simulink model "HANcoder_E407_DYS_MP"  (R2018b)
settings: Solver=FixedStepDiscrete  StartTime=0.0  StopTime=1  FixedStep=0.01  RelTol=1e-3
PreLoadFcn:
  | librarySetup
  | eval([bdroot,'_startup']) %Calling [modelName]_startup.m
values from neighbouring files (symbols this model uses):
  basic_cycle_duration_bc0 = TM_Reset_Board   + COMP_duration    (= 212)    [HANcoder_E407_DYS_MP_startup.m]
  basic_cycle_duration_bc1 = basic_cycle_duration_bc0    (= 212)    [HANcoder_E407_DYS_MP_startup.m]
  comm_delay_estimation1 = round(comm_delay_measured1*hardware_granularity/frequency_IRQ)    [HANcoder_E407_DYS_MP_startup.m]
  comm_delay_estimation2 = round(comm_delay_measured2*hardware_granularity/frequency_IRQ)    [HANcoder_E407_DYS_MP_startup.m]
  COMM_Phase1 = Simulink.Parameter    [HANcoder_E407_DYS_MP_startup.m]
  COMM_Phase2 = Simulink.Parameter    [HANcoder_E407_DYS_MP_startup.m]
  frequency_IRQ = 500    [HANcoder_E407_DYS_MP_startup.m]
  HantuneAngleSp = Simulink.Parameter    [HANcoder_E407_DYS_MP_startup.m]
  idle_time_init = basic_cycle_duration_bc0 + basic_cycle_duration_bc1    (= 424)    [HANcoder_E407_DYS_MP_startup.m]
  matrix_rows = 2    [HANcoder_E407_DYS_MP_startup.m]
  positionD = Simulink.Parameter    [HANcoder_E407_DYS_MP_startup.m]
  positionI = Simulink.Parameter    [HANcoder_E407_DYS_MP_startup.m]
  positionP = Simulink.Parameter    [HANcoder_E407_DYS_MP_startup.m]
undefined symbols (not defined in the file or in its folder): A1, CON2, CON4, D13, Dposition, Iposition, Pposition
libraries: HANcoder_STM32_Target x33, dspswit3 x16, simulink x2, simulink_extras x2, dspstat3 x1
(part 9 of 10)

== system HANcoder_E407_DYS_MP/HANcoder STM32 Target - E407-STM32 algorithm/4.TTA Can System/4.3 TTA System/4.3.3 Matrix Cycle Manager/4.3.3.1 Controller Matrix Cycle Truck Boards 1 2 and 3/4.3.3.1.2 controller basic cycle 0.2/Receive Truck 2 Board 2 Calc Steering Angle/Receive can message/CAN receive2 ==
  In1 : Inport
  Enabled Subsystem : Subsystem  TreatAsAtomicUnit=on
  S-Function : M-S-Function  FunctionName=sfcn_can_receive  Parameters=tsamp, canBus, outputNumber, dataType, byteOrder
  Term{3..9} (7 alike) : Terminator
  Out1 : Outport
  Out2 : Outport  Port=2
  wires:
  S-Function/9 -> Enabled Subsystem/8(In8)
  S-Function/4 -> Enabled Subsystem/3(In3)
  S-Function/5 -> Enabled Subsystem/4(In4)
  S-Function/8 -> Enabled Subsystem/7(In7)
  S-Function/7 -> Enabled Subsystem/6(In6)
  S-Function/6 -> Enabled Subsystem/5(In5)
  Enabled Subsystem/8(Out8) -> Term9/1
  Enabled Subsystem/7(Out7) -> Term8/1
  Enabled Subsystem/6(Out6) -> Term7/1
  Enabled Subsystem/5(Out5) -> Term6/1
  Enabled Subsystem/4(Out4) -> Term5/1
  Enabled Subsystem/3(Out3) -> Term4/1
  Enabled Subsystem/2(Out2) -> Term3/1
  Enabled Subsystem/1(Out1) -> Out2/1
  S-Function/3 -> Enabled Subsystem/2(In2)
  S-Function/2 -> Enabled Subsystem/1(In1)
  S-Function/1 -> Out1/1, Enabled Subsystem/Enable
  In1/1 -> S-Function/1

== system HANcoder_E407_DYS_MP/HANcoder STM32 Target - E407-STM32 algorithm/4.TTA Can System/4.3 TTA System/4.3.3 Matrix Cycle Manager/4.3.3.1 Controller Matrix Cycle Truck Boards 1 2 and 3/4.3.3.1.2 controller basic cycle 0.2/Receive Truck 3 Board 3 Calc Steering Angle/Receive can message/CAN receive ==
  In1 : Inport
  Enabled Subsystem : Subsystem  TreatAsAtomicUnit=on
  S-Function : M-S-Function  FunctionName=sfcn_can_receive  Parameters=tsamp, canBus, outputNumber, dataType, byteOrder
  Term{3..9} (7 alike) : Terminator
  Out1 : Outport
  Out2 : Outport  Port=2
  wires:
  S-Function/9 -> Enabled Subsystem/8(In8)
  S-Function/4 -> Enabled Subsystem/3(In3)
  S-Function/5 -> Enabled Subsystem/4(In4)
  S-Function/8 -> Enabled Subsystem/7(In7)
  S-Function/7 -> Enabled Subsystem/6(In6)
  S-Function/6 -> Enabled Subsystem/5(In5)
  Enabled Subsystem/8(Out8) -> Term9/1
  Enabled Subsystem/7(Out7) -> Term8/1
  Enabled Subsystem/6(Out6) -> Term7/1
  Enabled Subsystem/5(Out5) -> Term6/1
  Enabled Subsystem/4(Out4) -> Term5/1
  Enabled Subsystem/3(Out3) -> Term4/1
  Enabled Subsystem/2(Out2) -> Term3/1
  Enabled Subsystem/1(Out1) -> Out2/1
  S-Function/3 -> Enabled Subsystem/2(In2)
  S-Function/2 -> Enabled Subsystem/1(In1)
  S-Function/1 -> Out1/1, Enabled Subsystem/Enable
  In1/1 -> S-Function/1

== system HANcoder_E407_DYS_MP/HANcoder STM32 Target - E407-STM32 algorithm/4.TTA Can System/4.3 TTA System/4.3.3 Matrix Cycle Manager/4.3.3.1 Controller Matrix Cycle Truck Boards 1 2 and 3/4.3.3.1.2 controller basic cycle 0.2/Receive Truck 3 Board 3 Calc Steering Angle/Receive can message/CAN receive2 ==
  In1 : Inport
  Enabled Subsystem : Subsystem  TreatAsAtomicUnit=on
  S-Function : M-S-Function  FunctionName=sfcn_can_receive  Parameters=tsamp, canBus, outputNumber, dataType, byteOrder
  Term{3..9} (7 alike) : Terminator
  Out1 : Outport
  Out2 : Outport  Port=2
  wires:
  S-Function/9 -> Enabled Subsystem/8(In8)
  S-Function/4 -> Enabled Subsystem/3(In3)
  S-Function/5 -> Enabled Subsystem/4(In4)
  S-Function/8 -> Enabled Subsystem/7(In7)
  S-Function/7 -> Enabled Subsystem/6(In6)
  S-Function/6 -> Enabled Subsystem/5(In5)
  Enabled Subsystem/8(Out8) -> Term9/1
  Enabled Subsystem/7(Out7) -> Term8/1
  Enabled Subsystem/6(Out6) -> Term7/1
  Enabled Subsystem/5(Out5) -> Term6/1
  Enabled Subsystem/4(Out4) -> Term5/1
  Enabled Subsystem/3(Out3) -> Term4/1
  Enabled Subsystem/2(Out2) -> Term3/1
  Enabled Subsystem/1(Out1) -> Out2/1
  S-Function/3 -> Enabled Subsystem/2(In2)
  S-Function/2 -> Enabled Subsystem/1(In1)
  S-Function/1 -> Out1/1, Enabled Subsystem/Enable
  In1/1 -> S-Function/1

== system HANcoder_E407_DYS_MP/HANcoder STM32 Target - E407-STM32 algorithm/4.TTA Can System/4.3 TTA System/4.3.3 Matrix Cycle Manager/4.3.3.2 Controller Matrix Cycle_Board 4 and 5/controller basic cycle 0/Receive Timer can master message /Receive can message/CAN receive ==
  In1 : Inport
  Enabled Subsystem : Subsystem  TreatAsAtomicUnit=on
  S-Function : M-S-Function  FunctionName=sfcn_can_receive  Parameters=tsamp, canBus, outputNumber, dataType, byteOrder
  Term{3..9} (7 alike) : Terminator
  Out1 : Outport
  Out2 : Outport  Port=2
  wires:
  S-Function/9 -> Enabled Subsystem/8(In8)
  S-Function/4 -> Enabled Subsystem/3(In3)
  S-Function/5 -> Enabled Subsystem/4(In4)
  S-Function/8 -> Enabled Subsystem/7(In7)
  S-Function/7 -> Enabled Subsystem/6(In6)
  S-Function/6 -> Enabled Subsystem/5(In5)
  Enabled Subsystem/8(Out8) -> Term9/1
  Enabled Subsystem/7(Out7) -> Term8/1
  Enabled Subsystem/6(Out6) -> Term7/1
  Enabled Subsystem/5(Out5) -> Term6/1
  Enabled Subsystem/4(Out4) -> Term5/1
  Enabled Subsystem/3(Out3) -> Term4/1
  Enabled Subsystem/2(Out2) -> Term3/1
  Enabled Subsystem/1(Out1) -> Out2/1
  S-Function/3 -> Enabled Subsystem/2(In2)
  S-Function/2 -> Enabled Subsystem/1(In1)
  S-Function/1 -> Out1/1, Enabled Subsystem/Enable
  In1/1 -> S-Function/1

== system HANcoder_E407_DYS_MP/HANcoder STM32 Target - E407-STM32 algorithm/4.TTA Can System/4.3 TTA System/4.3.3 Matrix Cycle Manager/4.3.3.2 Controller Matrix Cycle_Board 4 and 5/controller basic cycle 0/Receive Timer can master message /Receive can message/CAN receive2 ==
  In1 : Inport
  Enabled Subsystem : Subsystem  TreatAsAtomicUnit=on
  S-Function : M-S-Function  FunctionName=sfcn_can_receive  Parameters=tsamp, canBus, outputNumber, dataType, byteOrder
  Term{3..9} (7 alike) : Terminator
  Out1 : Outport
  Out2 : Outport  Port=2
  wires:
  S-Function/9 -> Enabled Subsystem/8(In8)
  S-Function/4 -> Enabled Subsystem/3(In3)
  S-Function/5 -> Enabled Subsystem/4(In4)
  S-Function/8 -> Enabled Subsystem/7(In7)
  S-Function/7 -> Enabled Subsystem/6(In6)
  S-Function/6 -> Enabled Subsystem/5(In5)
  Enabled Subsystem/8(Out8) -> Term9/1
  Enabled Subsystem/7(Out7) -> Term8/1
  Enabled Subsystem/6(Out6) -> Term7/1
  Enabled Subsystem/5(Out5) -> Term6/1
  Enabled Subsystem/4(Out4) -> Term5/1
  Enabled Subsystem/3(Out3) -> Term4/1
  Enabled Subsystem/2(Out2) -> Term3/1
  Enabled Subsystem/1(Out1) -> Out2/1
  S-Function/3 -> Enabled Subsystem/2(In2)
  S-Function/2 -> Enabled Subsystem/1(In1)
  S-Function/1 -> Out1/1, Enabled Subsystem/Enable
  In1/1 -> S-Function/1

== system HANcoder_E407_DYS_MP/HANcoder STM32 Target - E407-STM32 algorithm/4.TTA Can System/4.3 TTA System/4.3.3 Matrix Cycle Manager/4.3.3.2 Controller Matrix Cycle_Board 4 and 5/controller basic cycle 0.2/Receive Trailer 1 board 4 input angel/Receive can message/CAN receive ==
  In1 : Inport
  Enabled Subsystem : Subsystem  TreatAsAtomicUnit=on
  S-Function : M-S-Function  FunctionName=sfcn_can_receive  Parameters=tsamp, canBus, outputNumber, dataType, byteOrder
  Term{3..9} (7 alike) : Terminator
  Out1 : Outport
  Out2 : Outport  Port=2
  wires:
  S-Function/9 -> Enabled Subsystem/8(In8)
  S-Function/4 -> Enabled Subsystem/3(In3)
  S-Function/5 -> Enabled Subsystem/4(In4)
  S-Function/8 -> Enabled Subsystem/7(In7)
  S-Function/7 -> Enabled Subsystem/6(In6)
  S-Function/6 -> Enabled Subsystem/5(In5)
  Enabled Subsystem/8(Out8) -> Term9/1
  Enabled Subsystem/7(Out7) -> Term8/1
  Enabled Subsystem/6(Out6) -> Term7/1
  Enabled Subsystem/5(Out5) -> Term6/1
  Enabled Subsystem/4(Out4) -> Term5/1
  Enabled Subsystem/3(Out3) -> Term4/1
  Enabled Subsystem/2(Out2) -> Term3/1
  Enabled Subsystem/1(Out1) -> Out2/1
  S-Function/3 -> Enabled Subsystem/2(In2)
  S-Function/2 -> Enabled Subsystem/1(In1)
  S-Function/1 -> Out1/1, Enabled Subsystem/Enable
  In1/1 -> S-Function/1

== system HANcoder_E407_DYS_MP/HANcoder STM32 Target - E407-STM32 algorithm/4.TTA Can System/4.3 TTA System/4.3.3 Matrix Cycle Manager/4.3.3.2 Controller Matrix Cycle_Board 4 and 5/controller basic cycle 0.2/Receive Trailer 1 board 4 input angel/Receive can message/CAN receive2 ==
  In1 : Inport
  Enabled Subsystem : Subsystem  TreatAsAtomicUnit=on
  S-Function : M-S-Function  FunctionName=sfcn_can_receive  Parameters=tsamp, canBus, outputNumber, dataType, byteOrder
  Term{3..9} (7 alike) : Terminator
  Out1 : Outport
  Out2 : Outport  Port=2
  wires:
  S-Function/9 -> Enabled Subsystem/8(In8)
  S-Function/4 -> Enabled Subsystem/3(In3)
  S-Function/5 -> Enabled Subsystem/4(In4)
  S-Function/8 -> Enabled Subsystem/7(In7)
  S-Function/7 -> Enabled Subsystem/6(In6)
  S-Function/6 -> Enabled Subsystem/5(In5)
  Enabled Subsystem/8(Out8) -> Term9/1
  Enabled Subsystem/7(Out7) -> Term8/1
  Enabled Subsystem/6(Out6) -> Term7/1
  Enabled Subsystem/5(Out5) -> Term6/1
  Enabled Subsystem/4(Out4) -> Term5/1
  Enabled Subsystem/3(Out3) -> Term4/1
  Enabled Subsystem/2(Out2) -> Term3/1
  Enabled Subsystem/1(Out1) -> Out2/1
  S-Function/3 -> Enabled Subsystem/2(In2)
  S-Function/2 -> Enabled Subsystem/1(In1)
  S-Function/1 -> Out1/1, Enabled Subsystem/Enable
  In1/1 -> S-Function/1

== system HANcoder_E407_DYS_MP/HANcoder STM32 Target - E407-STM32 algorithm/4.TTA Can System/4.3 TTA System/4.3.3 Matrix Cycle Manager/4.3.3.2 Controller Matrix Cycle_Board 4 and 5/controller basic cycle 0.2/Receive Trailer 2 board 5 input angel/Receive can message/CAN receive ==
  In1 : Inport
  Enabled Subsystem : Subsystem  TreatAsAtomicUnit=on
  S-Function : M-S-Function  FunctionName=sfcn_can_receive  Parameters=tsamp, canBus, outputNumber, dataType, byteOrder
  Term{3..9} (7 alike) : Terminator
  Out1 : Outport
  Out2 : Outport  Port=2
  wires:
  S-Function/9 -> Enabled Subsystem/8(In8)
  S-Function/4 -> Enabled Subsystem/3(In3)
  S-Function/5 -> Enabled Subsystem/4(In4)
  S-Function/8 -> Enabled Subsystem/7(In7)
  S-Function/7 -> Enabled Subsystem/6(In6)
  S-Function/6 -> Enabled Subsystem/5(In5)
  Enabled Subsystem/8(Out8) -> Term9/1
  Enabled Subsystem/7(Out7) -> Term8/1
  Enabled Subsystem/6(Out6) -> Term7/1
  Enabled Subsystem/5(Out5) -> Term6/1
  Enabled Subsystem/4(Out4) -> Term5/1
  Enabled Subsystem/3(Out3) -> Term4/1
  Enabled Subsystem/2(Out2) -> Term3/1
  Enabled Subsystem/1(Out1) -> Out2/1
  S-Function/3 -> Enabled Subsystem/2(In2)
  S-Function/2 -> Enabled Subsystem/1(In1)
  S-Function/1 -> Out1/1, Enabled Subsystem/Enable
  In1/1 -> S-Function/1

== system HANcoder_E407_DYS_MP/HANcoder STM32 Target - E407-STM32 algorithm/4.TTA Can System/4.3 TTA System/4.3.3 Matrix Cycle Manager/4.3.3.2 Controller Matrix Cycle_Board 4 and 5/controller basic cycle 0.2/Receive Trailer 2 board 5 input angel/Receive can message/CAN receive2 ==
  In1 : Inport
  Enabled Subsystem : Subsystem  TreatAsAtomicUnit=on
  S-Function : M-S-Function  FunctionName=sfcn_can_receive  Parameters=tsamp, canBus, outputNumber, dataType, byteOrder
  Term{3..9} (7 alike) : Terminator
  Out1 : Outport
  Out2 : Outport  Port=2
  wires:
  S-Function/9 -> Enabled Subsystem/8(In8)
  S-Function/4 -> Enabled Subsystem/3(In3)
  S-Function/5 -> Enabled Subsystem/4(In4)
  S-Function/8 -> Enabled Subsystem/7(In7)
  S-Function/7 -> Enabled Subsystem/6(In6)
  S-Function/6 -> Enabled Subsystem/5(In5)
  Enabled Subsystem/8(Out8) -> Term9/1
  Enabled Subsystem/7(Out7) -> Term8/1
  Enabled Subsystem/6(Out6) -> Term7/1
  Enabled Subsystem/5(Out5) -> Term6/1
  Enabled Subsystem/4(Out4) -> Term5/1
  Enabled Subsystem/3(Out3) -> Term4/1
  Enabled Subsystem/2(Out2) -> Term3/1
  Enabled Subsystem/1(Out1) -> Out2/1
  S-Function/3 -> Enabled Subsystem/2(In2)
  S-Function/2 -> Enabled Subsystem/1(In1)
  S-Function/1 -> Out1/1, Enabled Subsystem/Enable
  In1/1 -> S-Function/1

== system HANcoder_E407_DYS_MP/HANcoder STM32 Target - E407-STM32 algorithm/4.TTA Can System/4.3 TTA System/4.3.3 Matrix Cycle Manager/4.3.3.2 Controller Matrix Cycle_Board 4 and 5/controller basic cycle 0.2/Receive Truck 1 Board 1 Calc Steering Angle/Receive can message/CAN receive ==
  In1 : Inport
  Enabled Subsystem : Subsystem  TreatAsAtomicUnit=on
  S-Function : M-S-Function  FunctionName=sfcn_can_receive  Parameters=tsamp, canBus, outputNumber, dataType, byteOrder
  Term{3..9} (7 alike) : Terminator
  Out1 : Outport
  Out2 : Outport  Port=2
  wires:
  S-Function/9 -> Enabled Subsystem/8(In8)
  S-Function/4 -> Enabled Subsystem/3(In3)
  S-Function/5 -> Enabled Subsystem/4(In4)
  S-Function/8 -> Enabled Subsystem/7(In7)
  S-Function/7 -> Enabled Subsystem/6(In6)
  S-Function/6 -> Enabled Subsystem/5(In5)
  Enabled Subsystem/8(Out8) -> Term9/1
  Enabled Subsystem/7(Out7) -> Term8/1
  Enabled Subsystem/6(Out6) -> Term7/1
  Enabled Subsystem/5(Out5) -> Term6/1
  Enabled Subsystem/4(Out4) -> Term5/1
  Enabled Subsystem/3(Out3) -> Term4/1
  Enabled Subsystem/2(Out2) -> Term3/1
  Enabled Subsystem/1(Out1) -> Out2/1
  S-Function/3 -> Enabled Subsystem/2(In2)
  S-Function/2 -> Enabled Subsystem/1(In1)
  S-Function/1 -> Out1/1, Enabled Subsystem/Enable
  In1/1 -> S-Function/1

== system HANcoder_E407_DYS_MP/HANcoder STM32 Target - E407-STM32 algorithm/4.TTA Can System/4.3 TTA System/4.3.3 Matrix Cycle Manager/4.3.3.2 Controller Matrix Cycle_Board 4 and 5/controller basic cycle 0.2/Receive Truck 1 Board 1 Calc Steering Angle/Receive can message/CAN receive2 ==
  In1 : Inport
  Enabled Subsystem : Subsystem  TreatAsAtomicUnit=on
  S-Function : M-S-Function  FunctionName=sfcn_can_receive  Parameters=tsamp, canBus, outputNumber, dataType, byteOrder
  Term{3..9} (7 alike) : Terminator
  Out1 : Outport
  Out2 : Outport  Port=2
  wires:
  S-Function/9 -> Enabled Subsystem/8(In8)
  S-Function/4 -> Enabled Subsystem/3(In3)
  S-Function/5 -> Enabled Subsystem/4(In4)
  S-Function/8 -> Enabled Subsystem/7(In7)
  S-Function/7 -> Enabled Subsystem/6(In6)
  S-Function/6 -> Enabled Subsystem/5(In5)
  Enabled Subsystem/8(Out8) -> Term9/1
  Enabled Subsystem/7(Out7) -> Term8/1
  Enabled Subsystem/6(Out6) -> Term7/1
  Enabled Subsystem/5(Out5) -> Term6/1
  Enabled Subsystem/4(Out4) -> Term5/1
  Enabled Subsystem/3(Out3) -> Term4/1
  Enabled Subsystem/2(Out2) -> Term3/1
  Enabled Subsystem/1(Out1) -> Out2/1
  S-Function/3 -> Enabled Subsystem/2(In2)
  S-Function/2 -> Enabled Subsystem/1(In1)
  S-Function/1 -> Out1/1, Enabled Subsystem/Enable
  In1/1 -> S-Function/1

== system HANcoder_E407_DYS_MP/HANcoder STM32 Target - E407-STM32 algorithm/4.TTA Can System/4.3 TTA System/4.3.3 Matrix Cycle Manager/4.3.3.2 Controller Matrix Cycle_Board 4 and 5/controller basic cycle 0.2/Receive Truck 2 Board 2 Calc Steering Angle/Receive can message/CAN receive ==
  In1 : Inport
  Enabled Subsystem : Subsystem  TreatAsAtomicUnit=on
  S-Function : M-S-Function  FunctionName=sfcn_can_receive  Parameters=tsamp, canBus, outputNumber, dataType, byteOrder
  Term{3..9} (7 alike) : Terminator
  Out1 : Outport
  Out2 : Outport  Port=2
  wires:
  S-Function/9 -> Enabled Subsystem/8(In8)
  S-Function/4 -> Enabled Subsystem/3(In3)
  S-Function/5 -> Enabled Subsystem/4(In4)
  S-Function/8 -> Enabled Subsystem/7(In7)
  S-Function/7 -> Enabled Subsystem/6(In6)
  S-Function/6 -> Enabled Subsystem/5(In5)
  Enabled Subsystem/8(Out8) -> Term9/1
  Enabled Subsystem/7(Out7) -> Term8/1
  Enabled Subsystem/6(Out6) -> Term7/1
  Enabled Subsystem/5(Out5) -> Term6/1
  Enabled Subsystem/4(Out4) -> Term5/1
  Enabled Subsystem/3(Out3) -> Term4/1
  Enabled Subsystem/2(Out2) -> Term3/1
  Enabled Subsystem/1(Out1) -> Out2/1
  S-Function/3 -> Enabled Subsystem/2(In2)
  S-Function/2 -> Enabled Subsystem/1(In1)
  S-Function/1 -> Out1/1, Enabled Subsystem/Enable
  In1/1 -> S-Function/1

== system HANcoder_E407_DYS_MP/HANcoder STM32 Target - E407-STM32 algorithm/4.TTA Can System/4.3 TTA System/4.3.3 Matrix Cycle Manager/4.3.3.2 Controller Matrix Cycle_Board 4 and 5/controller basic cycle 0.2/Receive Truck 2 Board 2 Calc Steering Angle/Receive can message/CAN receive2 ==
  In1 : Inport
  Enabled Subsystem : Subsystem  TreatAsAtomicUnit=on
  S-Function : M-S-Function  FunctionName=sfcn_can_receive  Parameters=tsamp, canBus, outputNumber, dataType, byteOrder
  Term{3..9} (7 alike) : Terminator
  Out1 : Outport
  Out2 : Outport  Port=2
  wires:
  S-Function/9 -> Enabled Subsystem/8(In8)
  S-Function/4 -> Enabled Subsystem/3(In3)
  S-Function/5 -> Enabled Subsystem/4(In4)
  S-Function/8 -> Enabled Subsystem/7(In7)
  S-Function/7 -> Enabled Subsystem/6(In6)
  S-Function/6 -> Enabled Subsystem/5(In5)
  Enabled Subsystem/8(Out8) -> Term9/1
  Enabled Subsystem/7(Out7) -> Term8/1
  Enabled Subsystem/6(Out6) -> Term7/1
  Enabled Subsystem/5(Out5) -> Term6/1
  Enabled Subsystem/4(Out4) -> Term5/1
  Enabled Subsystem/3(Out3) -> Term4/1
  Enabled Subsystem/2(Out2) -> Term3/1
  Enabled Subsystem/1(Out1) -> Out2/1
  S-Function/3 -> Enabled Subsystem/2(In2)
  S-Function/2 -> Enabled Subsystem/1(In1)
  S-Function/1 -> Out1/1, Enabled Subsystem/Enable
  In1/1 -> S-Function/1

== system HANcoder_E407_DYS_MP/HANcoder STM32 Target - E407-STM32 algorithm/4.TTA Can System/4.3 TTA System/4.3.3 Matrix Cycle Manager/4.3.3.2 Controller Matrix Cycle_Board 4 and 5/controller basic cycle 0.2/Receive Truck 3 Board 3 Calc Steering Angle/Receive can message/CAN receive ==
  In1 : Inport
  Enabled Subsystem : Subsystem  TreatAsAtomicUnit=on
  S-Function : M-S-Function  FunctionName=sfcn_can_receive  Parameters=tsamp, canBus, outputNumber, dataType, byteOrder
  Term{3..9} (7 alike) : Terminator
  Out1 : Outport
  Out2 : Outport  Port=2
  wires:
  S-Function/9 -> Enabled Subsystem/8(In8)
  S-Function/4 -> Enabled Subsystem/3(In3)
  S-Function/5 -> Enabled Subsystem/4(In4)
  S-Function/8 -> Enabled Subsystem/7(In7)
  S-Function/7 -> Enabled Subsystem/6(In6)
  S-Function/6 -> Enabled Subsystem/5(In5)
  Enabled Subsystem/8(Out8) -> Term9/1
  Enabled Subsystem/7(Out7) -> Term8/1
  Enabled Subsystem/6(Out6) -> Term7/1
  Enabled Subsystem/5(Out5) -> Term6/1
  Enabled Subsystem/4(Out4) -> Term5/1
  Enabled Subsystem/3(Out3) -> Term4/1
  Enabled Subsystem/2(Out2) -> Term3/1
  Enabled Subsystem/1(Out1) -> Out2/1
  S-Function/3 -> Enabled Subsystem/2(In2)
  S-Function/2 -> Enabled Subsystem/1(In1)
  S-Function/1 -> Out1/1, Enabled Subsystem/Enable
  In1/1 -> S-Function/1

== system HANcoder_E407_DYS_MP/HANcoder STM32 Target - E407-STM32 algorithm/4.TTA Can System/4.3 TTA System/4.3.3 Matrix Cycle Manager/4.3.3.2 Controller Matrix Cycle_Board 4 and 5/controller basic cycle 0.2/Receive Truck 3 Board 3 Calc Steering Angle/Receive can message/CAN receive2 ==
  In1 : Inport
  Enabled Subsystem : Subsystem  TreatAsAtomicUnit=on
  S-Function : M-S-Function  FunctionName=sfcn_can_receive  Parameters=tsamp, canBus, outputNumber, dataType, byteOrder
  Term{3..9} (7 alike) : Terminator
  Out1 : Outport
  Out2 : Outport  Port=2
  wires:
  S-Function/9 -> Enabled Subsystem/8(In8)
  S-Function/4 -> Enabled Subsystem/3(In3)
  S-Function/5 -> Enabled Subsystem/4(In4)
  S-Function/8 -> Enabled Subsystem/7(In7)
  S-Function/7 -> Enabled Subsystem/6(In6)
  S-Function/6 -> Enabled Subsystem/5(In5)
  Enabled Subsystem/8(Out8) -> Term9/1
  Enabled Subsystem/7(Out7) -> Term8/1
  Enabled Subsystem/6(Out6) -> Term7/1
  Enabled Subsystem/5(Out5) -> Term6/1
  Enabled Subsystem/4(Out4) -> Term5/1
  Enabled Subsystem/3(Out3) -> Term4/1
  Enabled Subsystem/2(Out2) -> Term3/1
  Enabled Subsystem/1(Out1) -> Out2/1
  S-Function/3 -> Enabled Subsystem/2(In2)
  S-Function/2 -> Enabled Subsystem/1(In1)
  S-Function/1 -> Out1/1, Enabled Subsystem/Enable
  In1/1 -> S-Function/1

== system HANcoder_E407_DYS_MP/HANcoder STM32 Target - E407-STM32 algorithm/4.TTA Can System/4.3 TTA System/4.3.3 Matrix Cycle Manager/4.3.3.1 Controller Matrix Cycle Truck Boards 1 2 and 3/4.3.3.1.1 controller basic cycle 0.1/Receive Timer can master message /Receive can message/CAN receive/Enabled Subsystem ==
  In1 : Inport
  In2 : Inport  Port=2
  In3 : Inport  Port=3
  In4 : Inport  Port=4
  In5 : Inport  Port=5
  In6 : Inport  Port=6
  In7 : Inport  Port=7
  In8 : Inport  Port=8
  Enable : EnablePort
  Out1 : Outport
  Out2 : Outport  Port=2
  Out3 : Outport  Port=3
  Out4 : Outport  Port=4
  Out5 : Outport  Port=5
  Out6 : Outport  Port=6
  Out7 : Outport  Port=7
  Out8 : Outport  Port=8
  wires:
  In8/1 -> Out8/1
  In7/1 -> Out7/1
  In6/1 -> Out6/1
  In5/1 -> Out5/1
  In4/1 -> Out4/1
  In3/1 -> Out3/1
  In2/1 -> Out2/1
  In1/1 -> Out1/1

== system HANcoder_E407_DYS_MP/HANcoder STM32 Target - E407-STM32 algorithm/4.TTA Can System/4.3 TTA System/4.3.3 Matrix Cycle Manager/4.3.3.1 Controller Matrix Cycle Truck Boards 1 2 and 3/4.3.3.1.1 controller basic cycle 0.1/Receive Timer can master message /Receive can message/CAN receive2/Enabled Subsystem ==
  In1 : Inport
  In2 : Inport  Port=2
  In3 : Inport  Port=3
  In4 : Inport  Port=4
  In5 : Inport  Port=5
  In6 : Inport  Port=6
  In7 : Inport  Port=7
  In8 : Inport  Port=8
  Enable : EnablePort
  Out1 : Outport
  Out2 : Outport  Port=2
  Out3 : Outport  Port=3
  Out4 : Outport  Port=4
  Out5 : Outport  Port=5
  Out6 : Outport  Port=6
  Out7 : Outport  Port=7
  Out8 : Outport  Port=8
  wires:
  In8/1 -> Out8/1
  In7/1 -> Out7/1
  In6/1 -> Out6/1
  In5/1 -> Out5/1
  In4/1 -> Out4/1
  In3/1 -> Out3/1
  In2/1 -> Out2/1
  In1/1 -> Out1/1

== system HANcoder_E407_DYS_MP/HANcoder STM32 Target - E407-STM32 algorithm/4.TTA Can System/4.3 TTA System/4.3.3 Matrix Cycle Manager/4.3.3.1 Controller Matrix Cycle Truck Boards 1 2 and 3/4.3.3.1.1 controller basic cycle 0.1/Receive Timer can master message 1/Receive can message/CAN receive/Enabled Subsystem ==
  In1 : Inport
  In2 : Inport  Port=2
  In3 : Inport  Port=3
  In4 : Inport  Port=4
  In5 : Inport  Port=5
  In6 : Inport  Port=6
  In7 : Inport  Port=7
  In8 : Inport  Port=8
  Enable : EnablePort
  Out1 : Outport
  Out2 : Outport  Port=2
  Out3 : Outport  Port=3
  Out4 : Outport  Port=4
  Out5 : Outport  Port=5
  Out6 : Outport  Port=6
  Out7 : Outport  Port=7
  Out8 : Outport  Port=8
  wires:
  In8/1 -> Out8/1
  In7/1 -> Out7/1
  In6/1 -> Out6/1
  In5/1 -> Out5/1
  In4/1 -> Out4/1
  In3/1 -> Out3/1
  In2/1 -> Out2/1
  In1/1 -> Out1/1

== system HANcoder_E407_DYS_MP/HANcoder STM32 Target - E407-STM32 algorithm/4.TTA Can System/4.3 TTA System/4.3.3 Matrix Cycle Manager/4.3.3.1 Controller Matrix Cycle Truck Boards 1 2 and 3/4.3.3.1.1 controller basic cycle 0.1/Receive Timer can master message 1/Receive can message/CAN receive2/Enabled Subsystem ==
  In1 : Inport
  In2 : Inport  Port=2
  In3 : Inport  Port=3
  In4 : Inport  Port=4
  In5 : Inport  Port=5
  In6 : Inport  Port=6
  In7 : Inport  Port=7
  In8 : Inport  Port=8
  Enable : EnablePort
  Out1 : Outport
  Out2 : Outport  Port=2
  Out3 : Outport  Port=3
  Out4 : Outport  Port=4
  Out5 : Outport  Port=5
  Out6 : Outport  Port=6
  Out7 : Outport  Port=7
  Out8 : Outport  Port=8
  wires:
  In8/1 -> Out8/1
  In7/1 -> Out7/1
  In6/1 -> Out6/1
  In5/1 -> Out5/1
  In4/1 -> Out4/1
  In3/1 -> Out3/1
  In2/1 -> Out2/1
  In1/1 -> Out1/1

== system HANcoder_E407_DYS_MP/HANcoder STM32 Target - E407-STM32 algorithm/4.TTA Can System/4.3 TTA System/4.3.3 Matrix Cycle Manager/4.3.3.1 Controller Matrix Cycle Truck Boards 1 2 and 3/4.3.3.1.1 controller basic cycle 0.1/Receive Timer can master message 2/Receive can message/CAN receive/Enabled Subsystem ==
  In1 : Inport
  In2 : Inport  Port=2
  In3 : Inport  Port=3
  In4 : Inport  Port=4
  In5 : Inport  Port=5
  In6 : Inport  Port=6
  In7 : Inport  Port=7
  In8 : Inport  Port=8
  Enable : EnablePort
  Out1 : Outport
  Out2 : Outport  Port=2
  Out3 : Outport  Port=3
  Out4 : Outport  Port=4
  Out5 : Outport  Port=5
  Out6 : Outport  Port=6
  Out7 : Outport  Port=7
  Out8 : Outport  Port=8
  wires:
  In8/1 -> Out8/1
  In7/1 -> Out7/1
  In6/1 -> Out6/1
  In5/1 -> Out5/1
  In4/1 -> Out4/1
  In3/1 -> Out3/1
  In2/1 -> Out2/1
  In1/1 -> Out1/1

== system HANcoder_E407_DYS_MP/HANcoder STM32 Target - E407-STM32 algorithm/4.TTA Can System/4.3 TTA System/4.3.3 Matrix Cycle Manager/4.3.3.1 Controller Matrix Cycle Truck Boards 1 2 and 3/4.3.3.1.1 controller basic cycle 0.1/Receive Timer can master message 2/Receive can message/CAN receive2/Enabled Subsystem ==
  In1 : Inport
  In2 : Inport  Port=2
  In3 : Inport  Port=3
  In4 : Inport  Port=4
  In5 : Inport  Port=5
  In6 : Inport  Port=6
  In7 : Inport  Port=7
  In8 : Inport  Port=8
  Enable : EnablePort
  Out1 : Outport
  Out2 : Outport  Port=2
  Out3 : Outport  Port=3
  Out4 : Outport  Port=4
  Out5 : Outport  Port=5
  Out6 : Outport  Port=6
  Out7 : Outport  Port=7
  Out8 : Outport  Port=8
  wires:
  In8/1 -> Out8/1
  In7/1 -> Out7/1
  In6/1 -> Out6/1
  In5/1 -> Out5/1
  In4/1 -> Out4/1
  In3/1 -> Out3/1
  In2/1 -> Out2/1
  In1/1 -> Out1/1

== system HANcoder_E407_DYS_MP/HANcoder STM32 Target - E407-STM32 algorithm/4.TTA Can System/4.3 TTA System/4.3.3 Matrix Cycle Manager/4.3.3.1 Controller Matrix Cycle Truck Boards 1 2 and 3/4.3.3.1.1 controller basic cycle 0.1/Receive Timer can master message 3/Receive can message/CAN receive/Enabled Subsystem ==
  In1 : Inport
  In2 : Inport  Port=2
  In3 : Inport  Port=3
  In4 : Inport  Port=4
  In5 : Inport  Port=5
  In6 : Inport  Port=6
  In7 : Inport  Port=7
  In8 : Inport  Port=8
  Enable : EnablePort
  Out1 : Outport
  Out2 : Outport  Port=2
  Out3 : Outport  Port=3
  Out4 : Outport  Port=4
  Out5 : Outport  Port=5
  Out6 : Outport  Port=6
  Out7 : Outport  Port=7
  Out8 : Outport  Port=8
  wires:
  In8/1 -> Out8/1
  In7/1 -> Out7/1
  In6/1 -> Out6/1
  In5/1 -> Out5/1
  In4/1 -> Out4/1
  In3/1 -> Out3/1
  In2/1 -> Out2/1
  In1/1 -> Out1/1

== system HANcoder_E407_DYS_MP/HANcoder STM32 Target - E407-STM32 algorithm/4.TTA Can System/4.3 TTA System/4.3.3 Matrix Cycle Manager/4.3.3.1 Controller Matrix Cycle Truck Boards 1 2 and 3/4.3.3.1.1 controller basic cycle 0.1/Receive Timer can master message 3/Receive can message/CAN receive2/Enabled Subsystem ==
  In1 : Inport
  In2 : Inport  Port=2
  In3 : Inport  Port=3
  In4 : Inport  Port=4
  In5 : Inport  Port=5
  In6 : Inport  Port=6
  In7 : Inport  Port=7
  In8 : Inport  Port=8
  Enable : EnablePort
  Out1 : Outport
  Out2 : Outport  Port=2
  Out3 : Outport  Port=3
  Out4 : Outport  Port=4
  Out5 : Outport  Port=5
  Out6 : Outport  Port=6
  Out7 : Outport  Port=7
  Out8 : Outport  Port=8
  wires:
  In8/1 -> Out8/1
  In7/1 -> Out7/1
  In6/1 -> Out6/1
  In5/1 -> Out5/1
  In4/1 -> Out4/1
  In3/1 -> Out3/1
  In2/1 -> Out2/1
  In1/1 -> Out1/1

== system HANcoder_E407_DYS_MP/HANcoder STM32 Target - E407-STM32 algorithm/4.TTA Can System/4.3 TTA System/4.3.3 Matrix Cycle Manager/4.3.3.1 Controller Matrix Cycle Truck Boards 1 2 and 3/4.3.3.1.2 controller basic cycle 0.2/Receive Trailer 1 board 4 input angel/Receive can message/CAN receive/Enabled Subsystem ==
  In1 : Inport
  In2 : Inport  Port=2
  In3 : Inport  Port=3
  In4 : Inport  Port=4
  In5 : Inport  Port=5
  In6 : Inport  Port=6
  In7 : Inport  Port=7
  In8 : Inport  Port=8
  Enable : EnablePort
  Out1 : Outport
  Out2 : Outport  Port=2
  Out3 : Outport  Port=3
  Out4 : Outport  Port=4
  Out5 : Outport  Port=5
  Out6 : Outport  Port=6
  Out7 : Outport  Port=7
  Out8 : Outport  Port=8
  wires:
  In8/1 -> Out8/1
  In7/1 -> Out7/1
  In6/1 -> Out6/1
  In5/1 -> Out5/1
  In4/1 -> Out4/1
  In3/1 -> Out3/1
  In2/1 -> Out2/1
  In1/1 -> Out1/1

== system HANcoder_E407_DYS_MP/HANcoder STM32 Target - E407-STM32 algorithm/4.TTA Can System/4.3 TTA System/4.3.3 Matrix Cycle Manager/4.3.3.1 Controller Matrix Cycle Truck Boards 1 2 and 3/4.3.3.1.2 controller basic cycle 0.2/Receive Trailer 1 board 4 input angel/Receive can message/CAN receive2/Enabled Subsystem ==
  In1 : Inport
  In2 : Inport  Port=2
  In3 : Inport  Port=3
  In4 : Inport  Port=4
  In5 : Inport  Port=5
  In6 : Inport  Port=6
  In7 : Inport  Port=7
  In8 : Inport  Port=8
  Enable : EnablePort
  Out1 : Outport
  Out2 : Outport  Port=2
  Out3 : Outport  Port=3
  Out4 : Outport  Port=4
  Out5 : Outport  Port=5
  Out6 : Outport  Port=6
  Out7 : Outport  Port=7
  Out8 : Outport  Port=8
  wires:
  In8/1 -> Out8/1
  In7/1 -> Out7/1
  In6/1 -> Out6/1
  In5/1 -> Out5/1
  In4/1 -> Out4/1
  In3/1 -> Out3/1
  In2/1 -> Out2/1
  In1/1 -> Out1/1

== system HANcoder_E407_DYS_MP/HANcoder STM32 Target - E407-STM32 algorithm/4.TTA Can System/4.3 TTA System/4.3.3 Matrix Cycle Manager/4.3.3.1 Controller Matrix Cycle Truck Boards 1 2 and 3/4.3.3.1.2 controller basic cycle 0.2/Receive Trailer 2 board 5 input angel/Receive can message/CAN receive/Enabled Subsystem ==
  In1 : Inport
  In2 : Inport  Port=2
  In3 : Inport  Port=3
  In4 : Inport  Port=4
  In5 : Inport  Port=5
  In6 : Inport  Port=6
  In7 : Inport  Port=7
  In8 : Inport  Port=8
  Enable : EnablePort
  Out1 : Outport
  Out2 : Outport  Port=2
  Out3 : Outport  Port=3
  Out4 : Outport  Port=4
  Out5 : Outport  Port=5
  Out6 : Outport  Port=6
  Out7 : Outport  Port=7
  Out8 : Outport  Port=8
  wires:
  In8/1 -> Out8/1
  In7/1 -> Out7/1
  In6/1 -> Out6/1
  In5/1 -> Out5/1
  In4/1 -> Out4/1
  In3/1 -> Out3/1
  In2/1 -> Out2/1
  In1/1 -> Out1/1

== system HANcoder_E407_DYS_MP/HANcoder STM32 Target - E407-STM32 algorithm/4.TTA Can System/4.3 TTA System/4.3.3 Matrix Cycle Manager/4.3.3.1 Controller Matrix Cycle Truck Boards 1 2 and 3/4.3.3.1.2 controller basic cycle 0.2/Receive Trailer 2 board 5 input angel/Receive can message/CAN receive2/Enabled Subsystem ==
  In1 : Inport
  In2 : Inport  Port=2
  In3 : Inport  Port=3
  In4 : Inport  Port=4
  In5 : Inport  Port=5
  In6 : Inport  Port=6
  In7 : Inport  Port=7
  In8 : Inport  Port=8
  Enable : EnablePort
  Out1 : Outport
  Out2 : Outport  Port=2
  Out3 : Outport  Port=3
  Out4 : Outport  Port=4
  Out5 : Outport  Port=5
  Out6 : Outport  Port=6
  Out7 : Outport  Port=7
  Out8 : Outport  Port=8
  wires:
  In8/1 -> Out8/1
  In7/1 -> Out7/1
  In6/1 -> Out6/1
  In5/1 -> Out5/1
  In4/1 -> Out4/1
  In3/1 -> Out3/1
  In2/1 -> Out2/1
  In1/1 -> Out1/1

== system HANcoder_E407_DYS_MP/HANcoder STM32 Target - E407-STM32 algorithm/4.TTA Can System/4.3 TTA System/4.3.3 Matrix Cycle Manager/4.3.3.1 Controller Matrix Cycle Truck Boards 1 2 and 3/4.3.3.1.2 controller basic cycle 0.2/Receive Truck 1 Board 1 Calc Steering Angle/Receive can message/CAN receive/Enabled Subsystem ==
  In1 : Inport
  In2 : Inport  Port=2
  In3 : Inport  Port=3
  In4 : Inport  Port=4
  In5 : Inport  Port=5
  In6 : Inport  Port=6
  In7 : Inport  Port=7
  In8 : Inport  Port=8
  Enable : EnablePort
  Out1 : Outport
  Out2 : Outport  Port=2
  Out3 : Outport  Port=3
  Out4 : Outport  Port=4
  Out5 : Outport  Port=5
  Out6 : Outport  Port=6
  Out7 : Outport  Port=7
  Out8 : Outport  Port=8
  wires:
  In8/1 -> Out8/1
  In7/1 -> Out7/1
  In6/1 -> Out6/1
  In5/1 -> Out5/1
  In4/1 -> Out4/1
  In3/1 -> Out3/1
  In2/1 -> Out2/1
  In1/1 -> Out1/1

== system HANcoder_E407_DYS_MP/HANcoder STM32 Target - E407-STM32 algorithm/4.TTA Can System/4.3 TTA System/4.3.3 Matrix Cycle Manager/4.3.3.1 Controller Matrix Cycle Truck Boards 1 2 and 3/4.3.3.1.2 controller basic cycle 0.2/Receive Truck 1 Board 1 Calc Steering Angle/Receive can message/CAN receive2/Enabled Subsystem ==
  In1 : Inport
  In2 : Inport  Port=2
  In3 : Inport  Port=3
  In4 : Inport  Port=4
  In5 : Inport  Port=5
  In6 : Inport  Port=6
  In7 : Inport  Port=7
  In8 : Inport  Port=8
  Enable : EnablePort
  Out1 : Outport
  Out2 : Outport  Port=2
  Out3 : Outport  Port=3
  Out4 : Outport  Port=4
  Out5 : Outport  Port=5
  Out6 : Outport  Port=6
  Out7 : Outport  Port=7
  Out8 : Outport  Port=8
  wires:
  In8/1 -> Out8/1
  In7/1 -> Out7/1
  In6/1 -> Out6/1
  In5/1 -> Out5/1
  In4/1 -> Out4/1
  In3/1 -> Out3/1
  In2/1 -> Out2/1
  In1/1 -> Out1/1

== system HANcoder_E407_DYS_MP/HANcoder STM32 Target - E407-STM32 algorithm/4.TTA Can System/4.3 TTA System/4.3.3 Matrix Cycle Manager/4.3.3.1 Controller Matrix Cycle Truck Boards 1 2 and 3/4.3.3.1.2 controller basic cycle 0.2/Receive Truck 1 Board 1 Calc Steering Angle1/Receive can message/CAN receive/Enabled Subsystem ==
  In1 : Inport
  In2 : Inport  Port=2
  In3 : Inport  Port=3
  In4 : Inport  Port=4
  In5 : Inport  Port=5
  In6 : Inport  Port=6
  In7 : Inport  Port=7
  In8 : Inport  Port=8
  Enable : EnablePort
  Out1 : Outport
  Out2 : Outport  Port=2
  Out3 : Outport  Port=3
  Out4 : Outport  Port=4
  Out5 : Outport  Port=5
  Out6 : Outport  Port=6
  Out7 : Outport  Port=7
  Out8 : Outport  Port=8
  wires:
  In8/1 -> Out8/1
  In7/1 -> Out7/1
  In6/1 -> Out6/1
  In5/1 -> Out5/1
  In4/1 -> Out4/1
  In3/1 -> Out3/1
  In2/1 -> Out2/1
  In1/1 -> Out1/1

== system HANcoder_E407_DYS_MP/HANcoder STM32 Target - E407-STM32 algorithm/4.TTA Can System/4.3 TTA System/4.3.3 Matrix Cycle Manager/4.3.3.1 Controller Matrix Cycle Truck Boards 1 2 and 3/4.3.3.1.2 controller basic cycle 0.2/Receive Truck 1 Board 1 Calc Steering Angle1/Receive can message/CAN receive2/Enabled Subsystem ==
  In1 : Inport
  In2 : Inport  Port=2
  In3 : Inport  Port=3
  In4 : Inport  Port=4
  In5 : Inport  Port=5
  In6 : Inport  Port=6
  In7 : Inport  Port=7
  In8 : Inport  Port=8
  Enable : EnablePort
  Out1 : Outport
  Out2 : Outport  Port=2
  Out3 : Outport  Port=3
  Out4 : Outport  Port=4
  Out5 : Outport  Port=5
  Out6 : Outport  Port=6
  Out7 : Outport  Port=7
  Out8 : Outport  Port=8
  wires:
  In8/1 -> Out8/1
  In7/1 -> Out7/1
  In6/1 -> Out6/1
  In5/1 -> Out5/1
  In4/1 -> Out4/1
  In3/1 -> Out3/1
  In2/1 -> Out2/1
  In1/1 -> Out1/1

== system HANcoder_E407_DYS_MP/HANcoder STM32 Target - E407-STM32 algorithm/4.TTA Can System/4.3 TTA System/4.3.3 Matrix Cycle Manager/4.3.3.1 Controller Matrix Cycle Truck Boards 1 2 and 3/4.3.3.1.2 controller basic cycle 0.2/Receive Truck 1 Board 1 Calc Steering Angle2/Receive can message/CAN receive/Enabled Subsystem ==
  In1 : Inport
  In2 : Inport  Port=2
  In3 : Inport  Port=3
  In4 : Inport  Port=4
  In5 : Inport  Port=5
  In6 : Inport  Port=6
  In7 : Inport  Port=7
  In8 : Inport  Port=8
  Enable : EnablePort
  Out1 : Outport
  Out2 : Outport  Port=2
  Out3 : Outport  Port=3
  Out4 : Outport  Port=4
  Out5 : Outport  Port=5
  Out6 : Outport  Port=6
  Out7 : Outport  Port=7
  Out8 : Outport  Port=8
  wires:
  In8/1 -> Out8/1
  In7/1 -> Out7/1
  In6/1 -> Out6/1
  In5/1 -> Out5/1
  In4/1 -> Out4/1
  In3/1 -> Out3/1
  In2/1 -> Out2/1
  In1/1 -> Out1/1

== system HANcoder_E407_DYS_MP/HANcoder STM32 Target - E407-STM32 algorithm/4.TTA Can System/4.3 TTA System/4.3.3 Matrix Cycle Manager/4.3.3.1 Controller Matrix Cycle Truck Boards 1 2 and 3/4.3.3.1.2 controller basic cycle 0.2/Receive Truck 1 Board 1 Calc Steering Angle2/Receive can message/CAN receive2/Enabled Subsystem ==
  In1 : Inport
  In2 : Inport  Port=2
  In3 : Inport  Port=3
  In4 : Inport  Port=4
  In5 : Inport  Port=5
  In6 : Inport  Port=6
  In7 : Inport  Port=7
  In8 : Inport  Port=8
  Enable : EnablePort
  Out1 : Outport
  Out2 : Outport  Port=2
  Out3 : Outport  Port=3
  Out4 : Outport  Port=4
  Out5 : Outport  Port=5
  Out6 : Outport  Port=6
  Out7 : Outport  Port=7
  Out8 : Outport  Port=8
  wires:
  In8/1 -> Out8/1
  In7/1 -> Out7/1
  In6/1 -> Out6/1
  In5/1 -> Out5/1
  In4/1 -> Out4/1
  In3/1 -> Out3/1
  In2/1 -> Out2/1
  In1/1 -> Out1/1

== system HANcoder_E407_DYS_MP/HANcoder STM32 Target - E407-STM32 algorithm/4.TTA Can System/4.3 TTA System/4.3.3 Matrix Cycle Manager/4.3.3.1 Controller Matrix Cycle Truck Boards 1 2 and 3/4.3.3.1.2 controller basic cycle 0.2/Receive Truck 1 Board 1 Calc Steering Angle3/Receive can message/CAN receive/Enabled Subsystem ==
  In1 : Inport
  In2 : Inport  Port=2
  In3 : Inport  Port=3
  In4 : Inport  Port=4
  In5 : Inport  Port=5
  In6 : Inport  Port=6
  In7 : Inport  Port=7
  In8 : Inport  Port=8
  Enable : EnablePort
  Out1 : Outport
  Out2 : Outport  Port=2
  Out3 : Outport  Port=3
  Out4 : Outport  Port=4
  Out5 : Outport  Port=5
  Out6 : Outport  Port=6
  Out7 : Outport  Port=7
  Out8 : Outport  Port=8
  wires:
  In8/1 -> Out8/1
  In7/1 -> Out7/1
  In6/1 -> Out6/1
  In5/1 -> Out5/1
  In4/1 -> Out4/1
  In3/1 -> Out3/1
  In2/1 -> Out2/1
  In1/1 -> Out1/1

== system HANcoder_E407_DYS_MP/HANcoder STM32 Target - E407-STM32 algorithm/4.TTA Can System/4.3 TTA System/4.3.3 Matrix Cycle Manager/4.3.3.1 Controller Matrix Cycle Truck Boards 1 2 and 3/4.3.3.1.2 controller basic cycle 0.2/Receive Truck 1 Board 1 Calc Steering Angle3/Receive can message/CAN receive2/Enabled Subsystem ==
  In1 : Inport
  In2 : Inport  Port=2
  In3 : Inport  Port=3
  In4 : Inport  Port=4
  In5 : Inport  Port=5
  In6 : Inport  Port=6
  In7 : Inport  Port=7
  In8 : Inport  Port=8
  Enable : EnablePort
  Out1 : Outport
  Out2 : Outport  Port=2
  Out3 : Outport  Port=3
  Out4 : Outport  Port=4
  Out5 : Outport  Port=5
  Out6 : Outport  Port=6
  Out7 : Outport  Port=7
  Out8 : Outport  Port=8
  wires:
  In8/1 -> Out8/1
  In7/1 -> Out7/1
  In6/1 -> Out6/1
  In5/1 -> Out5/1
  In4/1 -> Out4/1
  In3/1 -> Out3/1
  In2/1 -> Out2/1
  In1/1 -> Out1/1

== system HANcoder_E407_DYS_MP/HANcoder STM32 Target - E407-STM32 algorithm/4.TTA Can System/4.3 TTA System/4.3.3 Matrix Cycle Manager/4.3.3.1 Controller Matrix Cycle Truck Boards 1 2 and 3/4.3.3.1.2 controller basic cycle 0.2/Receive Truck 2 Board 2 Calc Steering Angle/Receive can message/CAN receive/Enabled Subsystem ==
  In1 : Inport
  In2 : Inport  Port=2
  In3 : Inport  Port=3
  In4 : Inport  Port=4
  In5 : Inport  Port=5
  In6 : Inport  Port=6
  In7 : Inport  Port=7
  In8 : Inport  Port=8
  Enable : EnablePort
  Out1 : Outport
  Out2 : Outport  Port=2
  Out3 : Outport  Port=3
  Out4 : Outport  Port=4
  Out5 : Outport  Port=5
  Out6 : Outport  Port=6
  Out7 : Outport  Port=7
  Out8 : Outport  Port=8
  wires:
  In8/1 -> Out8/1
  In7/1 -> Out7/1
  In6/1 -> Out6/1
  In5/1 -> Out5/1
  In4/1 -> Out4/1
  In3/1 -> Out3/1
  In2/1 -> Out2/1
  In1/1 -> Out1/1

== system HANcoder_E407_DYS_MP/HANcoder STM32 Target - E407-STM32 algorithm/4.TTA Can System/4.3 TTA System/4.3.3 Matrix Cycle Manager/4.3.3.1 Controller Matrix Cycle Truck Boards 1 2 and 3/4.3.3.1.2 controller basic cycle 0.2/Receive Truck 2 Board 2 Calc Steering Angle/Receive can message/CAN receive2/Enabled Subsystem ==
  In1 : Inport
  In2 : Inport  Port=2
  In3 : Inport  Port=3
  In4 : Inport  Port=4
  In5 : Inport  Port=5
  In6 : Inport  Port=6
  In7 : Inport  Port=7
  In8 : Inport  Port=8
  Enable : EnablePort
  Out1 : Outport
  Out2 : Outport  Port=2
  Out3 : Outport  Port=3
  Out4 : Outport  Port=4
  Out5 : Outport  Port=5
  Out6 : Outport  Port=6
  Out7 : Outport  Port=7
  Out8 : Outport  Port=8
  wires:
  In8/1 -> Out8/1
  In7/1 -> Out7/1
  In6/1 -> Out6/1
  In5/1 -> Out5/1
  In4/1 -> Out4/1
  In3/1 -> Out3/1
  In2/1 -> Out2/1
  In1/1 -> Out1/1

== system HANcoder_E407_DYS_MP/HANcoder STM32 Target - E407-STM32 algorithm/4.TTA Can System/4.3 TTA System/4.3.3 Matrix Cycle Manager/4.3.3.1 Controller Matrix Cycle Truck Boards 1 2 and 3/4.3.3.1.2 controller basic cycle 0.2/Receive Truck 3 Board 3 Calc Steering Angle/Receive can message/CAN receive/Enabled Subsystem ==
  In1 : Inport
  In2 : Inport  Port=2
  In3 : Inport  Port=3
  In4 : Inport  Port=4
  In5 : Inport  Port=5
  In6 : Inport  Port=6
  In7 : Inport  Port=7
  In8 : Inport  Port=8
  Enable : EnablePort
  Out1 : Outport
  Out2 : Outport  Port=2
  Out3 : Outport  Port=3
  Out4 : Outport  Port=4
  Out5 : Outport  Port=5
  Out6 : Outport  Port=6
  Out7 : Outport  Port=7
  Out8 : Outport  Port=8
  wires:
  In8/1 -> Out8/1
  In7/1 -> Out7/1
  In6/1 -> Out6/1
  In5/1 -> Out5/1
  In4/1 -> Out4/1
  In3/1 -> Out3/1
  In2/1 -> Out2/1
  In1/1 -> Out1/1

== system HANcoder_E407_DYS_MP/HANcoder STM32 Target - E407-STM32 algorithm/4.TTA Can System/4.3 TTA System/4.3.3 Matrix Cycle Manager/4.3.3.1 Controller Matrix Cycle Truck Boards 1 2 and 3/4.3.3.1.2 controller basic cycle 0.2/Receive Truck 3 Board 3 Calc Steering Angle/Receive can message/CAN receive2/Enabled Subsystem ==
  In1 : Inport
  In2 : Inport  Port=2
  In3 : Inport  Port=3
  In4 : Inport  Port=4
  In5 : Inport  Port=5
  In6 : Inport  Port=6
  In7 : Inport  Port=7
  In8 : Inport  Port=8
  Enable : EnablePort
  Out1 : Outport
  Out2 : Outport  Port=2
  Out3 : Outport  Port=3
  Out4 : Outport  Port=4
  Out5 : Outport  Port=5
  Out6 : Outport  Port=6
  Out7 : Outport  Port=7
  Out8 : Outport  Port=8
  wires:
  In8/1 -> Out8/1
  In7/1 -> Out7/1
  In6/1 -> Out6/1
  In5/1 -> Out5/1
  In4/1 -> Out4/1
  In3/1 -> Out3/1
  In2/1 -> Out2/1
  In1/1 -> Out1/1

== system HANcoder_E407_DYS_MP/HANcoder STM32 Target - E407-STM32 algorithm/4.TTA Can System/4.3 TTA System/4.3.3 Matrix Cycle Manager/4.3.3.2 Controller Matrix Cycle_Board 4 and 5/controller basic cycle 0/Receive Timer can master message /Receive can message/CAN receive/Enabled Subsystem ==
  In1 : Inport
  In2 : Inport  Port=2
  In3 : Inport  Port=3
  In4 : Inport  Port=4
  In5 : Inport  Port=5
  In6 : Inport  Port=6
  In7 : Inport  Port=7
  In8 : Inport  Port=8
  Enable : EnablePort
  Out1 : Outport
  Out2 : Outport  Port=2
  Out3 : Outport  Port=3
  Out4 : Outport  Port=4
  Out5 : Outport  Port=5
  Out6 : Outport  Port=6
  Out7 : Outport  Port=7
  Out8 : Outport  Port=8
  wires:
  In8/1 -> Out8/1
  In7/1 -> Out7/1
  In6/1 -> Out6/1
  In5/1 -> Out5/1
  In4/1 -> Out4/1
  In3/1 -> Out3/1
  In2/1 -> Out2/1
  In1/1 -> Out1/1

== system HANcoder_E407_DYS_MP/HANcoder STM32 Target - E407-STM32 algorithm/4.TTA Can System/4.3 TTA System/4.3.3 Matrix Cycle Manager/4.3.3.2 Controller Matrix Cycle_Board 4 and 5/controller basic cycle 0/Receive Timer can master message /Receive can message/CAN receive2/Enabled Subsystem ==
  In1 : Inport
  In2 : Inport  Port=2
  In3 : Inport  Port=3
  In4 : Inport  Port=4
  In5 : Inport  Port=5
  In6 : Inport  Port=6
  In7 : Inport  Port=7
  In8 : Inport  Port=8
  Enable : EnablePort
  Out1 : Outport
  Out2 : Outport  Port=2
  Out3 : Outport  Port=3
  Out4 : Outport  Port=4
  Out5 : Outport  Port=5
  Out6 : Outport  Port=6
  Out7 : Outport  Port=7
  Out8 : Outport  Port=8
  wires:
  In8/1 -> Out8/1
  In7/1 -> Out7/1
  In6/1 -> Out6/1
  In5/1 -> Out5/1
  In4/1 -> Out4/1
  In3/1 -> Out3/1
  In2/1 -> Out2/1
  In1/1 -> Out1/1

== system HANcoder_E407_DYS_MP/HANcoder STM32 Target - E407-STM32 algorithm/4.TTA Can System/4.3 TTA System/4.3.3 Matrix Cycle Manager/4.3.3.2 Controller Matrix Cycle_Board 4 and 5/controller basic cycle 0.2/Receive Trailer 1 board 4 input angel/Receive can message/CAN receive/Enabled Subsystem ==
  In1 : Inport
  In2 : Inport  Port=2
  In3 : Inport  Port=3
  In4 : Inport  Port=4
  In5 : Inport  Port=5
  In6 : Inport  Port=6
  In7 : Inport  Port=7
  In8 : Inport  Port=8
  Enable : EnablePort
  Out1 : Outport
  Out2 : Outport  Port=2
  Out3 : Outport  Port=3
  Out4 : Outport  Port=4
  Out5 : Outport  Port=5
  Out6 : Outport  Port=6
  Out7 : Outport  Port=7
  Out8 : Outport  Port=8
  wires:
  In8/1 -> Out8/1
  In7/1 -> Out7/1
  In6/1 -> Out6/1
  In5/1 -> Out5/1
  In4/1 -> Out4/1
  In3/1 -> Out3/1
  In2/1 -> Out2/1
  In1/1 -> Out1/1

== system HANcoder_E407_DYS_MP/HANcoder STM32 Target - E407-STM32 algorithm/4.TTA Can System/4.3 TTA System/4.3.3 Matrix Cycle Manager/4.3.3.2 Controller Matrix Cycle_Board 4 and 5/controller basic cycle 0.2/Receive Trailer 1 board 4 input angel/Receive can message/CAN receive2/Enabled Subsystem ==
  In1 : Inport
  In2 : Inport  Port=2
  In3 : Inport  Port=3
  In4 : Inport  Port=4
  In5 : Inport  Port=5
  In6 : Inport  Port=6
  In7 : Inport  Port=7
  In8 : Inport  Port=8
  Enable : EnablePort
  Out1 : Outport
  Out2 : Outport  Port=2
  Out3 : Outport  Port=3
  Out4 : Outport  Port=4
  Out5 : Outport  Port=5
  Out6 : Outport  Port=6
  Out7 : Outport  Port=7
  Out8 : Outport  Port=8
  wires:
  In8/1 -> Out8/1
  In7/1 -> Out7/1
  In6/1 -> Out6/1
  In5/1 -> Out5/1
  In4/1 -> Out4/1
  In3/1 -> Out3/1
  In2/1 -> Out2/1
  In1/1 -> Out1/1

== system HANcoder_E407_DYS_MP/HANcoder STM32 Target - E407-STM32 algorithm/4.TTA Can System/4.3 TTA System/4.3.3 Matrix Cycle Manager/4.3.3.2 Controller Matrix Cycle_Board 4 and 5/controller basic cycle 0.2/Receive Trailer 2 board 5 input angel/Receive can message/CAN receive/Enabled Subsystem ==
  In1 : Inport
  In2 : Inport  Port=2
  In3 : Inport  Port=3
  In4 : Inport  Port=4
  In5 : Inport  Port=5
  In6 : Inport  Port=6
  In7 : Inport  Port=7
  In8 : Inport  Port=8
  Enable : EnablePort
  Out1 : Outport
  Out2 : Outport  Port=2
  Out3 : Outport  Port=3
  Out4 : Outport  Port=4
  Out5 : Outport  Port=5
  Out6 : Outport  Port=6
  Out7 : Outport  Port=7
  Out8 : Outport  Port=8
  wires:
  In8/1 -> Out8/1
  In7/1 -> Out7/1
  In6/1 -> Out6/1
  In5/1 -> Out5/1
  In4/1 -> Out4/1
  In3/1 -> Out3/1
  In2/1 -> Out2/1
  In1/1 -> Out1/1

== system HANcoder_E407_DYS_MP/HANcoder STM32 Target - E407-STM32 algorithm/4.TTA Can System/4.3 TTA System/4.3.3 Matrix Cycle Manager/4.3.3.2 Controller Matrix Cycle_Board 4 and 5/controller basic cycle 0.2/Receive Trailer 2 board 5 input angel/Receive can message/CAN receive2/Enabled Subsystem ==
  In1 : Inport
  In2 : Inport  Port=2
  In3 : Inport  Port=3
  In4 : Inport  Port=4
  In5 : Inport  Port=5
  In6 : Inport  Port=6
  In7 : Inport  Port=7
  In8 : Inport  Port=8
  Enable : EnablePort
  Out1 : Outport
  Out2 : Outport  Port=2
  Out3 : Outport  Port=3
  Out4 : Outport  Port=4
  Out5 : Outport  Port=5
  Out6 : Outport  Port=6
  Out7 : Outport  Port=7
  Out8 : Outport  Port=8
  wires:
  In8/1 -> Out8/1
  In7/1 -> Out7/1
  In6/1 -> Out6/1
  In5/1 -> Out5/1
  In4/1 -> Out4/1
  In3/1 -> Out3/1
  In2/1 -> Out2/1
  In1/1 -> Out1/1

== system HANcoder_E407_DYS_MP/HANcoder STM32 Target - E407-STM32 algorithm/4.TTA Can System/4.3 TTA System/4.3.3 Matrix Cycle Manager/4.3.3.2 Controller Matrix Cycle_Board 4 and 5/controller basic cycle 0.2/Receive Truck 1 Board 1 Calc Steering Angle/Receive can message/CAN receive/Enabled Subsystem ==
  In1 : Inport
  In2 : Inport  Port=2
  In3 : Inport  Port=3
  In4 : Inport  Port=4
  In5 : Inport  Port=5
  In6 : Inport  Port=6
  In7 : Inport  Port=7
  In8 : Inport  Port=8
  Enable : EnablePort
  Out1 : Outport
  Out2 : Outport  Port=2
  Out3 : Outport  Port=3
  Out4 : Outport  Port=4
  Out5 : Outport  Port=5
  Out6 : Outport  Port=6
  Out7 : Outport  Port=7
  Out8 : Outport  Port=8
  wires:
  In8/1 -> Out8/1
  In7/1 -> Out7/1
  In6/1 -> Out6/1
  In5/1 -> Out5/1
  In4/1 -> Out4/1
  In3/1 -> Out3/1
  In2/1 -> Out2/1
  In1/1 -> Out1/1

== system HANcoder_E407_DYS_MP/HANcoder STM32 Target - E407-STM32 algorithm/4.TTA Can System/4.3 TTA System/4.3.3 Matrix Cycle Manager/4.3.3.2 Controller Matrix Cycle_Board 4 and 5/controller basic cycle 0.2/Receive Truck 1 Board 1 Calc Steering Angle/Receive can message/CAN receive2/Enabled Subsystem ==
  In1 : Inport
  In2 : Inport  Port=2
  In3 : Inport  Port=3
  In4 : Inport  Port=4
  In5 : Inport  Port=5
  In6 : Inport  Port=6
  In7 : Inport  Port=7
  In8 : Inport  Port=8
  Enable : EnablePort
  Out1 : Outport
  Out2 : Outport  Port=2
  Out3 : Outport  Port=3
  Out4 : Outport  Port=4
  Out5 : Outport  Port=5
  Out6 : Outport  Port=6
  Out7 : Outport  Port=7
  Out8 : Outport  Port=8
  wires:
  In8/1 -> Out8/1
  In7/1 -> Out7/1
  In6/1 -> Out6/1
  In5/1 -> Out5/1
  In4/1 -> Out4/1
  In3/1 -> Out3/1
  In2/1 -> Out2/1
  In1/1 -> Out1/1

== system HANcoder_E407_DYS_MP/HANcoder STM32 Target - E407-STM32 algorithm/4.TTA Can System/4.3 TTA System/4.3.3 Matrix Cycle Manager/4.3.3.2 Controller Matrix Cycle_Board 4 and 5/controller basic cycle 0.2/Receive Truck 2 Board 2 Calc Steering Angle/Receive can message/CAN receive/Enabled Subsystem ==
  In1 : Inport
  In2 : Inport  Port=2
  In3 : Inport  Port=3
  In4 : Inport  Port=4
  In5 : Inport  Port=5
  In6 : Inport  Port=6
  In7 : Inport  Port=7
  In8 : Inport  Port=8
  Enable : EnablePort
  Out1 : Outport
  Out2 : Outport  Port=2
  Out3 : Outport  Port=3
  Out4 : Outport  Port=4
  Out5 : Outport  Port=5
  Out6 : Outport  Port=6
  Out7 : Outport  Port=7
  Out8 : Outport  Port=8
  wires:
  In8/1 -> Out8/1
  In7/1 -> Out7/1
  In6/1 -> Out6/1
  In5/1 -> Out5/1
  In4/1 -> Out4/1
  In3/1 -> Out3/1
  In2/1 -> Out2/1
  In1/1 -> Out1/1
